simulink model "trenl"  (R2023a)
settings: Solver=FixedStepDiscrete  StartTime=0.0  StopTime=10.0  RelTol=1e-3
values from neighbouring files (symbols this model uses):
  Am = 40    [main.m]
  NP = 0.9    [main.m]
  R = a    [main.m]
  repeated_seq = zeros(Ns + 1, 2)    [main.m]
  to = round(rand * 100)    [main.m]
  Ts = 1/200    (= 0.005)    [main.m]
libraries: commanapbnd3 x2, simulink x1
settings Model: Creator=kelfi  LastModifiedBy=kelfi

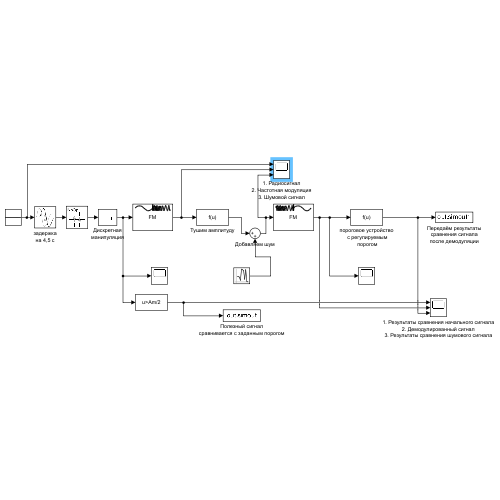
[thumbnail: Simulink's stored preview of the top-level diagram]
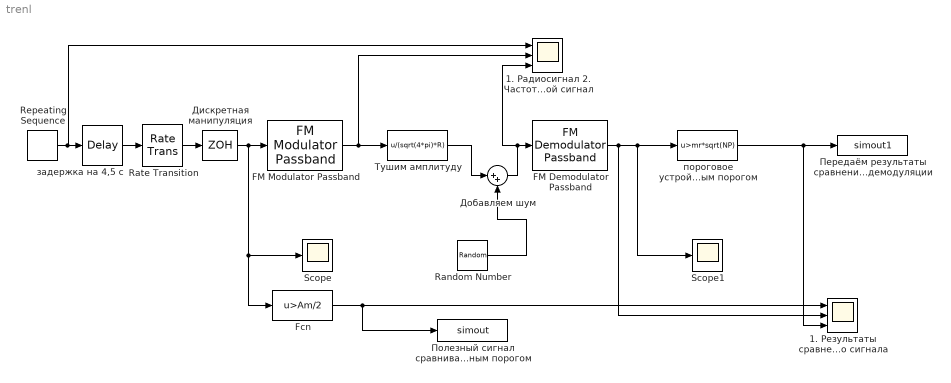
== system trenl ==
  1. Радиосигнал 2. Частотная модуляция 3. Шумовой сигнал : Scope  NumInputPorts=3
  1. Результаты сравнения начального сигнала 2. Демодулированный сигнал 3. Результаты сравнения шумового сигнала : Scope  NumInputPorts=3
  FM Demodulator Passband : commanapbnd3/FM Demodulator Passband  Fc=Hz  Ph=0  Kc=10  Ho=10
  FM Modulator Passband : commanapbnd3/FM Modulator Passband  Fc=Hz  Ph=0  Kc=10
  Fcn : Fcn  Expr=u>Am/2
  Random Number : RandomNumber  Variance=NP  Seed=to  SampleTime=Ts
  Rate Transition : RateTransition  OutPortSampleTimeOpt=Inherit  OutPortSampleTime=Ts
  Repeating Sequence : simulink/Sources/Repeating Sequence  rep_seq_t=repeated_seq(:, 1)  rep_seq_y=repeated_seq(:, 2)
  Scope : Scope
  Scope1 : Scope
  Дискретная манипуляция : ZeroOrderHold  SampleTime=-1
  Добавляем шум : Sum  Inputs=|++
  Передаём результаты сравнения сигнала после демодуляции : ToWorkspace  VariableName=simout1  SampleTime=Ts
      settings: Save2DSignal=2-D array (concatenate along first dimension)
  Полезный сигнал сравнивается с заданным порогом : ToWorkspace  VariableName=simout  SampleTime=Ts
      settings: Save2DSignal=2-D array (concatenate along first dimension)
  Тушим амплитуду : Fcn  Expr=u/(sqrt(4*pi)*R)
  задержка на 4,5 с : TransportDelay  InitialOutput=Am  BufferSize=10240
  пороговое устройство с регулируемым порогом : Fcn  Expr=u>mr*sqrt(NP)
  wires:
  FM Modulator Passband/1 -> Тушим амплитуду/1, 1. Радиосигнал 2. Частотная модуляция 3. Шумовой сигнал/2
  Random Number/1 -> Добавляем шум/2
  пороговое устройство с регулируемым порогом/1 -> Передаём результаты сравнения сигнала после демодуляции/1, 1. Результаты сравнения начального сигнала 2. Демодулированный сигнал 3. Результаты сравнения шумового сигнала/3
  Fcn/1 -> 1. Результаты сравнения начального сигнала 2. Демодулированный сигнал 3. Результаты сравнения шумового сигнала/1, Полезный сигнал сравнивается с заданным порогом/1
  Тушим амплитуду/1 -> Добавляем шум/1
  задержка на 4,5 с/1 -> Rate Transition/1
  Добавляем шум/1 -> 1. Радиосигнал 2. Частотная модуляция 3. Шумовой сигнал/3, FM Demodulator Passband/1
  Repeating Sequence/1 -> 1. Радиосигнал 2. Частотная модуляция 3. Шумовой сигнал/1, задержка на 4,5 с/1
  FM Demodulator Passband/1 -> Scope1/1, пороговое устройство с регулируемым порогом/1, 1. Результаты сравнения начального сигнала 2. Демодулированный сигнал 3. Результаты сравнения шумового сигнала/2
  Дискретная манипуляция/1 -> Fcn/1, Scope/1, FM Modulator Passband/1
  Rate Transition/1 -> Дискретная манипуляция/1
